simulink model "EDIF_start_up_v03"  (R2021b)
settings: Solver=FixedStepDiscrete  StartTime=0.0  StopTime=Inf  FixedStep=Ts  RelTol=1e-3  EnableMultiTasking=on
undefined symbols (not defined in the file or in its folder): Down, GPTRIP1SEL, Ts, TZ1, Up
libraries: c280xlib x6, svdutilitieslib x4, c2837xDlib x3, c2802xlib x2, simulink_extras x2, simulink x1, c2000sensorslib x1
settings Model: ExtModeTrigDuration=8  Creator=whendrix  LastModifiedBy=whendrix
settings SolverCC: AlgebraicLoopSolver=TrustRegion  AutoInsertRateTranBlk=on
settings DataIOCC: ReturnWorkspaceOutputs=off
settings OptimizationCC: DefaultUnderspecifiedDataType=single  EnhancedBackFolding=on  PassReuseOutputArgsAs=Individual arguments  MaxStackSize=1024  OptimizeBlockOrder=speed  DifferentSizesBufferReuse=on  OptimizationCustomize=off  DenormalBehavior=FlushToZero  EfficientTunableParamExpr=on
settings DebuggingCC: ParameterOverflowMsg=warning  ParameterPrecisionLossMsg=none  ParameterTunabilityLossMsg=error  SFMachineParentedDataDiag=warning  ArithmeticOperatorsInVariantConditions=warning
settings HardwareCC: ProdBitPerChar=16  ProdBitPerInt=16  ProdBitPerPointer=32  ProdBitPerSizeT=32  ProdBitPerPtrDiffT=32  ProdLargestAtomicInteger=Integer  ProdLargestAtomicFloat=None  ProdWordSize=16  ProdLongLongMode=on  ProdHWDeviceType=Texas Instruments->C2000
settings SFSimCC: MATLABDynamicMemAlloc=off  CustomCodeUndefinedFunction=UseInterfaceOnly
settings RTWCC: Description=Embedded Coder  SystemTargetFile=ert.tlc  HardwareBoard=TI Delfino F28379D LaunchPad  TemplateMakefile=ert_default_tmf  Toolchain=Texas Instruments Code Composer Studio (C2000)  IncludeHyperlinkInReport=on
settings CodeAppCC: ForceParamTrailComments=on  IgnoreCustomStorageClasses=off  OperatorAnnotations=on  SimulinkDataObjDesc=on  SFDataObjDesc=on  InsertBlockDesc=on
settings ERTTargetCC: CodeReplacementLibrary=TI C28x  ExtModeTransport=4  ExtModeStaticAlloc=on  ExtModeMexFile=ext_xcp  ExtModeIntrfLevel=Level2 - Open

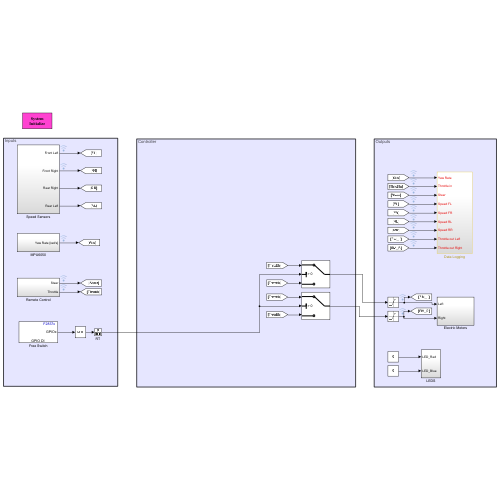
[thumbnail: Simulink's stored preview of the top-level diagram]
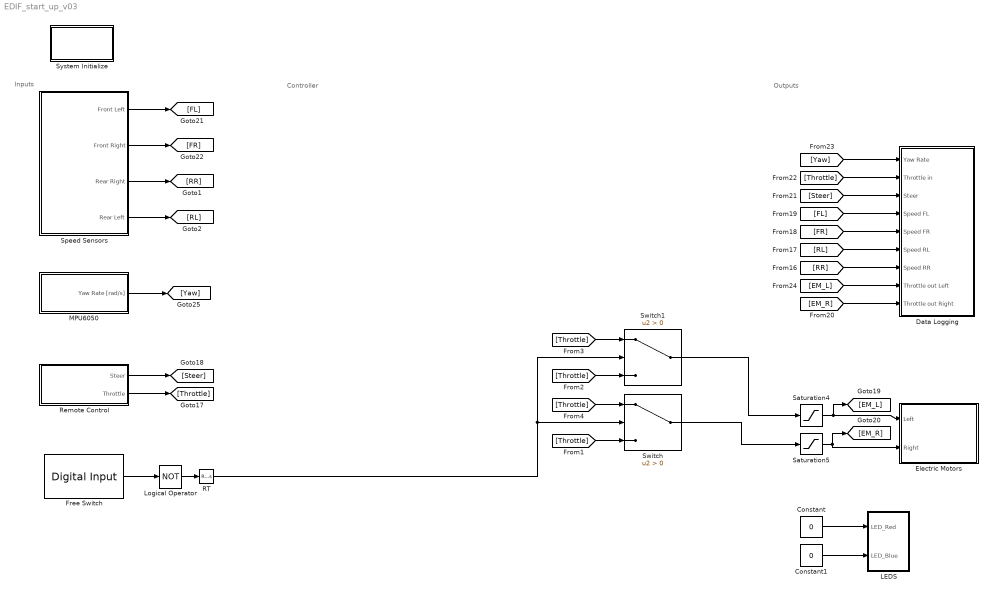
== system EDIF_start_up_v03 ==
  note: Controller
  note: Inputs
  note: Outputs
  Constant : Constant  Value=0
  Constant1 : Constant  Value=0
  Data Logging : Subsystem
  Electric Motors : Subsystem
  Free Switch : c2837xDlib/Digital Input  GPIO_Number=GPIO120~GPIO127  GPIO_Bit0=off  GPIO_Bit1=off  GPIO_Bit2=on  GPIO_Bit3=off  GPIO_Bit4=off  GPIO_Bit5=off  GPIO_Bit6=off  GPIO_Bit7=off  sampleTime=0.1  dataType=auto  GPIO_Bit0_Qualification=Sync to SYSCLKOUT  GPIO_Bit1_Qualification=Sync to SYSCLKOUT  GPIO_Bit2_Qualification=Sync to SYSCLKOUT  GPIO_Bit3_Qualification=Sync to SYSCLKOUT  GPIO_Bit4_Qualification=Sync to SYSCLKOUT  GPIO_Bit5_Qualification=Sync to SYSCLKOUT  GPIO_Bit6_Qualification=Sync to SYSCLKOUT  GPIO_Bit7_Qualification=Sync to SYSCLKOUT  Qualification_Period=-1
      settings: SourceProductBaseCode=TIC2000
  LEDS : Subsystem
  Logical Operator : Logic  Operator=NOT  AllPortsSameDT=off  OutDataTypeStr=boolean
  MPU6050 : Subsystem
  RT : RateTransition  OutPortSampleTime=0.005
  Remote Control : Subsystem
  Saturation4 : Saturate  UpperLimit=100  LowerLimit=20
  Saturation5 : Saturate  UpperLimit=100  LowerLimit=20
  Speed Sensors : Subsystem
  Switch : Switch  Criteria=u2 > Threshold  OutDataTypeStr=single
  Switch1 : Switch  Criteria=u2 > Threshold  OutDataTypeStr=single
  System Initialize : Subsystem  mask(System Initialize){ShowInLibBrowser=0}
      mask prompts: ShowInLibBrowser "Simulink:masks:CustCodeMaskParam1_MP"
      settings: CopyFcn=cccopyfcn(gcb)  OpenFcn=ccopenfcn('System Initialize Function')
      mask Help: eval('feval(''rtwprivate'',''rtwhelpview'',''rtw_sys_initialize_block'')');
      mask Display: disp('System\nInitialize');
  wires:
  MPU6050/1(Yaw Rate [rad/s]) -> [Yaw]
  Speed Sensors/1(Front Left) -> [FL]
  Saturation5/1 -> [EM_R], Electric Motors/2(Right)
  Saturation4/1 -> [EM_L], Electric Motors/1(Left)
  Speed Sensors/2(Front Right) -> [FR]
  Constant/1 -> LEDS/1(LED_Red)
  Remote Control/1(Steer) -> [Steer]
  [Yaw] -> Data Logging/1(Yaw Rate)
  [Throttle] -> Data Logging/2(Throttle in)
  [Steer] -> Data Logging/3(Steer)
  [FL] -> Data Logging/4(Speed FL)
  [FR] -> Data Logging/5(Speed FR)
  [RL] -> Data Logging/6(Speed RL)
  [RR] -> Data Logging/7(Speed RR)
  [EM_L] -> Data Logging/8(Throttle out Left)
  [EM_R] -> Data Logging/9(Throttle out Right)
  Speed Sensors/3(Rear Right) -> [RR]
  Speed Sensors/4(Rear Left) -> [RL]
  Remote Control/2(Throttle) -> [Throttle]
  Switch/1 -> Saturation5/1
  Switch1/1 -> Saturation4/1
  RT/1 -> Switch1/2, Switch/2
  [Throttle] -> Switch/3
  [Throttle] -> Switch1/3
  Logical Operator/1 -> RT/1
  Constant1/1 -> LEDS/2(LED_Blue)
  Free Switch/1 -> Logical Operator/1
  [Throttle] -> Switch1/1
  [Throttle] -> Switch/1

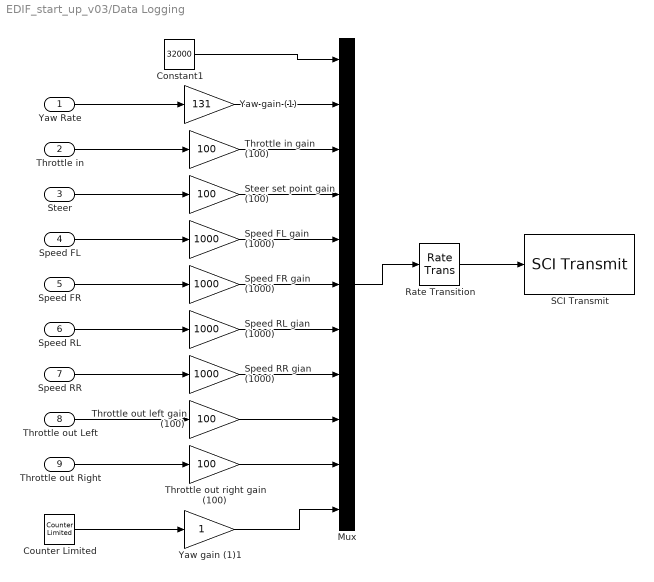
== system EDIF_start_up_v03/Data Logging ==
  Yaw Rate : Inport
  Throttle in : Inport  Port=2
  Steer : Inport  Port=3
  Speed FL : Inport  Port=4
  Speed FR : Inport  Port=5
  Speed RL : Inport  Port=6
  Speed RR : Inport  Port=7
  Throttle out Left : Inport  Port=8
  Throttle out Right : Inport  Port=9
  Constant1 : Constant  Value=32000  OutDataTypeStr=int16  SampleTime=0.005
  Counter Limited : simulink/Sources/Counter Limited  uplimit=30000  tsamp=Ts
  Mux : Mux  Inputs=11
  Rate Transition : RateTransition  OutPortSampleTime=0.01
  SCI Transmit : c280xlib/SCI Transmit  sciModule=B  dataHead=''  dataTail=''  postInterrupt=off  numFifo=1
  Speed FL gain (1000) : Gain  Gain=1000  OutDataTypeStr=int16
  Speed FR gain (1000) : Gain  Gain=1000  OutDataTypeStr=int16
  Speed RL gian (1000) : Gain  Gain=1000  OutDataTypeStr=int16
  Speed RR gian (1000) : Gain  Gain=1000  OutDataTypeStr=int16
  Steer set point gain (100) : Gain  Gain=100  OutDataTypeStr=int16
  Throttle in gain (100) : Gain  Gain=100  OutDataTypeStr=int16
  Throttle out left gain (100) : Gain  Gain=100  OutDataTypeStr=int16
  Throttle out right gain (100) : Gain  Gain=100  OutDataTypeStr=int16
  Yaw gain (1) : Gain  Gain=131  OutDataTypeStr=int16
  Yaw gain (1)1 : Gain  OutDataTypeStr=int16
  wires:
  Rate Transition/1 -> SCI Transmit/1
  Throttle out Left/1 -> Throttle out left gain (100)/1
  Speed RR/1 -> Speed RR gian (1000)/1
  Speed FR/1 -> Speed FR gain (1000)/1
  Speed RL/1 -> Speed RL gian (1000)/1
  Speed FL/1 -> Speed FL gain (1000)/1
  Throttle out Right/1 -> Throttle out right gain (100)/1
  Yaw Rate/1 -> Yaw gain (1)/1
  Throttle in/1 -> Throttle in gain (100)/1
  Steer/1 -> Steer set point gain (100)/1
  Throttle out right gain (100)/1 -> Mux/10
  Throttle out left gain (100)/1 -> Mux/9
  Speed RR gian (1000)/1 -> Mux/8
  Speed RL gian (1000)/1 -> Mux/7
  Speed FR gain (1000)/1 -> Mux/6
  Speed FL gain (1000)/1 -> Mux/5
  Steer set point gain (100)/1 -> Mux/4
  Throttle in gain (100)/1 -> Mux/3
  Yaw gain (1)/1 -> Mux/2
  Mux/1 -> Rate Transition/1
  Constant1/1 -> Mux/1
  Counter Limited/1 -> Yaw gain (1)1/1
  Yaw gain (1)1/1 -> Mux/11

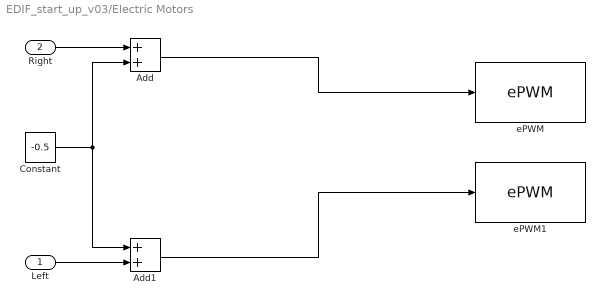
== system EDIF_start_up_v03/Electric Motors ==
  Left : Inport
  Right : Inport  Port=2
  Add : Sum
  Add1 : Sum
  Constant : Constant  Value=-0.5
  ePWM : c2802xlib/ePWM  PwmType=C2000_Type4  useModule=ePWM4  ePWMxLINKTBPRD=Not Linked  periodUnits=Clock cycles  timerSource=Specify via dialog  timerPeriod_clk=2000  timerPeriod_sec=0.0001  tbshadow=Counter equals to zero  countingMode=Up-Down  phaseActiveEnable=Disable  phaseDirection=Count down after sync  phaseActive=0  synchronizationEnable=off  dcaevt1Sync=off  dcbevt1Sync=off  synchronizationOption=Disable  perSynchronizationOption=Counter equals to period (CTR=PRD)  clockPrescale=1  HSclockPrescale=1  enswap=off  ePWMxAStatus=on  ePWMxAactionLogic1=Set  ePWMxAactionLogic2=Clear  ePWMxAactionLogic3=Clear  ePWMxAactionLogic4=Set  ePWMxAactionLogic5=Do nothing  ePWMxAactionLogic6=Do nothing  ePWMxACSFenable=off  ePWMxACSFvalue=Forcing disable  ePWMxASFreload=Zero  ePWMxBStatus=off  ePWMxBactionLogic1=Set  ePWMxBactionLogic2=Clear  ePWMxBactionLogic3=Do nothing  ePWMxBactionLogic4=Do nothing  ePWMxBactionLogic5=Clear  ePWMxBactionLogic6=Set  ePWMxBCSFenable=off  ePWMxBCSFvalue=Forcing disable  ePWMxBSFreload=Zero  ePWNxBOutWay=off  ePWMxLINKCMPA=Not Linked  CMPAUnits=Percentages  CMPASource=Input port  CMPAValue_per=50  CMPAValue_clk=32000  enCMPAshadow=Counter equals to zero (CTR=Zero)  ePWMxLINKCMPB=Not Linked  CMPBUnits=Clock cycles  CMPBSource=Specify via dialog  CMPBValue_per=50  CMPBValue_clk=32000  enCMPBshadow=Counter equals to zero (CTR=Zero)  ePWMxLINKCMPC=Not Linked  CMPCUnits=Clock cycles  CMPCSource=Specify via dialog  CMPCValue_per=50  CMPCValue_clk=32000  enCMPCshadow=Counter equals to zero (CTR=Zero)  ePWMxLINKCMPD=Not Linked  CMPDUnits=Clock cycles  CMPDSource=Specify via dialog  CMPDValue_per=50  CMPDValue_clk=32000  enCMPDshadow=Counter equals to zero (CTR=Zero)  enableDBePWMxA=off  enableDBePWMxB=off  enhalfcycle=off  DBpolarity=Active high (AH)  DBedgeDelay=Positive  DBSource_ePWMxA=ePWMxA  DBSource_ePWMxB=ePWMxA  DBPeriodUnits=Clock cycles  DBperiodSource=Specify via dialog  REDperiod=0  FEDperiod=0  REDperiod_sec=0  FEDperiod_sec=0  LoadModeDBRED=Immediate without using shadow  LoadModeDBFED=Immediate without using shadow  adcstartModuleA=off  adcrequestEventA=First event  adcstartEventA=Digital Compare Module A Event 1 start of conversion (DCAEVT1.soc)  adcstartEventA_type2=Counter equals to zero (CTR=Zero)  adcstartModuleB=off  adcrequestEventB=First event  adcstartEventB=Counter equals to zero (CTR=Zero)  adcstartEventB_type2=Counter equals to zero (CTR=Zero)  intEn=off  intPrd=First event  intSel=Counter equals to zero (CTR=Zero)  intSel_type2=Counter equals to zero (CTR=Zero)  hrpe=off  enHRPWM=off  HRPWM_LoadMode=Counter equals to period (CTR=PRD)  HRPWM_CTLMode=Duty or Period control mode  HRPWM_EDGMode=Both edge  hrpeb=off  enHRPWMB=off  HRPWM_LoadModeB=Counter equals to zero (CTR=ZERO)  HRPWM_CTLModeB=Duty or Period control mode  HRPWM_EDGModeB=Both edge  enHRDBRED=off  enHRDBFED=off  enSFO=on  enautoconv=on  chopperEnable=off  chopperFrequency=1  chopperFirstwidth=1  chopperDuty=12.5%  tripZonesource=Specify via dialog  tzselOSHT1=off  tzselOSHT2=off  tzselOSHT3=off  tzselOSHDCAEV1=off  tzselOSHDCBEV1=off  tzselCBC1=off  tzselCBC2=off  tzselCBC3=off  tzselCBCDCAEV2=off  tzselCBCDCBEV2=off  tzselOSHT4=off  tzselOSHT5=off  tzselOSHT6=off  tzselCBC4=off  tzselCBC5=off  tzselCBC6=off  enTzOstIntr=off  enTzCbcIntr=off  enTzDCAEVT1Intr=off  enTzDCAEVT2Intr=off  enTzDCBEVT1Intr=off  enTzDCBEVT2Intr=off  ePWMxAforced=No action  ePWMxBforced=No action  DCAEVT1forced=No action  DCBEVT1forced=No action  DCAEVT2forced=No action  DCBEVT2forced=No action  dcah=Trip Zone 1 input (TZ1)  dcal=Trip Zone 2 input (TZ2)  dcbh=Trip Zone 1 input (TZ1)  dcbl=Trip Zone 2 input (TZ2)  dcah_type2=GPTRIP1SEL/(TZ1)  dcal_type2=GPTRIP1SEL/(TZ1)  dcbh_type2=GPTRIP1SEL/(TZ1)  dcbl_type2=GPTRIP1SEL/(TZ1)  gendcaevt1=Event disabled  gendcaevt2=Event disabled  gendcbevt1=Event disabled  gendcbevt2=Event disabled  dcaevt1src=DCAEVT1 with sync  dcaevt2src=DCAEVT2 with sync  dcbevt1src=DCBEVT1 with sync  dcbevt2src=DCBEVT2 with sync  pulsesel=Counter equals to zero (CTR=Zero)  blankinv=off  blankoffset=0  blankwidth=0  evsrcsel=Filtered version of DCAEVT1 (DCAEVT1FILT)  encape=off
  ePWM1 : c2802xlib/ePWM  PwmType=C2000_Type4  useModule=ePWM5  ePWMxLINKTBPRD=Not Linked  periodUnits=Clock cycles  timerSource=Specify via dialog  timerPeriod_clk=2000  timerPeriod_sec=0.0001  tbshadow=Counter equals to zero  countingMode=Up-Down  phaseActiveEnable=Disable  phaseDirection=Count down after sync  phaseActive=0  synchronizationEnable=off  dcaevt1Sync=off  dcbevt1Sync=off  synchronizationOption=Disable  perSynchronizationOption=Counter equals to period (CTR=PRD)  clockPrescale=1  HSclockPrescale=1  enswap=off  ePWMxAStatus=on  ePWMxAactionLogic1=Set  ePWMxAactionLogic2=Clear  ePWMxAactionLogic3=Clear  ePWMxAactionLogic4=Set  ePWMxAactionLogic5=Do nothing  ePWMxAactionLogic6=Do nothing  ePWMxACSFenable=off  ePWMxACSFvalue=Forcing disable  ePWMxASFreload=Zero  ePWMxBStatus=off  ePWMxBactionLogic1=Set  ePWMxBactionLogic2=Clear  ePWMxBactionLogic3=Do nothing  ePWMxBactionLogic4=Do nothing  ePWMxBactionLogic5=Clear  ePWMxBactionLogic6=Set  ePWMxBCSFenable=off  ePWMxBCSFvalue=Forcing disable  ePWMxBSFreload=Zero  ePWNxBOutWay=off  ePWMxLINKCMPA=Not Linked  CMPAUnits=Percentages  CMPASource=Input port  CMPAValue_per=50  CMPAValue_clk=32000  enCMPAshadow=Counter equals to zero (CTR=Zero)  ePWMxLINKCMPB=Not Linked  CMPBUnits=Clock cycles  CMPBSource=Specify via dialog  CMPBValue_per=50  CMPBValue_clk=32000  enCMPBshadow=Counter equals to zero (CTR=Zero)  ePWMxLINKCMPC=Not Linked  CMPCUnits=Clock cycles  CMPCSource=Specify via dialog  CMPCValue_per=50  CMPCValue_clk=32000  enCMPCshadow=Counter equals to zero (CTR=Zero)  ePWMxLINKCMPD=Not Linked  CMPDUnits=Clock cycles  CMPDSource=Specify via dialog  CMPDValue_per=50  CMPDValue_clk=32000  enCMPDshadow=Counter equals to zero (CTR=Zero)  enableDBePWMxA=off  enableDBePWMxB=off  enhalfcycle=off  DBpolarity=Active high (AH)  DBedgeDelay=Positive  DBSource_ePWMxA=ePWMxA  DBSource_ePWMxB=ePWMxA  DBPeriodUnits=Clock cycles  DBperiodSource=Specify via dialog  REDperiod=0  FEDperiod=0  REDperiod_sec=0  FEDperiod_sec=0  LoadModeDBRED=Immediate without using shadow  LoadModeDBFED=Immediate without using shadow  adcstartModuleA=off  adcrequestEventA=First event  adcstartEventA=Digital Compare Module A Event 1 start of conversion (DCAEVT1.soc)  adcstartEventA_type2=Counter equals to zero (CTR=Zero)  adcstartModuleB=off  adcrequestEventB=First event  adcstartEventB=Counter equals to zero (CTR=Zero)  adcstartEventB_type2=Counter equals to zero (CTR=Zero)  intEn=off  intPrd=First event  intSel=Counter equals to zero (CTR=Zero)  intSel_type2=Counter equals to zero (CTR=Zero)  hrpe=off  enHRPWM=off  HRPWM_LoadMode=Counter equals to period (CTR=PRD)  HRPWM_CTLMode=Duty or Period control mode  HRPWM_EDGMode=Both edge  hrpeb=off  enHRPWMB=off  HRPWM_LoadModeB=Counter equals to zero (CTR=ZERO)  HRPWM_CTLModeB=Duty or Period control mode  HRPWM_EDGModeB=Both edge  enHRDBRED=off  enHRDBFED=off  enSFO=on  enautoconv=on  chopperEnable=off  chopperFrequency=1  chopperFirstwidth=1  chopperDuty=12.5%  tripZonesource=Specify via dialog  tzselOSHT1=off  tzselOSHT2=off  tzselOSHT3=off  tzselOSHDCAEV1=off  tzselOSHDCBEV1=off  tzselCBC1=off  tzselCBC2=off  tzselCBC3=off  tzselCBCDCAEV2=off  tzselCBCDCBEV2=off  tzselOSHT4=off  tzselOSHT5=off  tzselOSHT6=off  tzselCBC4=off  tzselCBC5=off  tzselCBC6=off  enTzOstIntr=off  enTzCbcIntr=off  enTzDCAEVT1Intr=off  enTzDCAEVT2Intr=off  enTzDCBEVT1Intr=off  enTzDCBEVT2Intr=off  ePWMxAforced=No action  ePWMxBforced=No action  DCAEVT1forced=No action  DCBEVT1forced=No action  DCAEVT2forced=No action  DCBEVT2forced=No action  dcah=Trip Zone 1 input (TZ1)  dcal=Trip Zone 2 input (TZ2)  dcbh=Trip Zone 1 input (TZ1)  dcbl=Trip Zone 2 input (TZ2)  dcah_type2=GPTRIP1SEL/(TZ1)  dcal_type2=GPTRIP1SEL/(TZ1)  dcbh_type2=GPTRIP1SEL/(TZ1)  dcbl_type2=GPTRIP1SEL/(TZ1)  gendcaevt1=Event disabled  gendcaevt2=Event disabled  gendcbevt1=Event disabled  gendcbevt2=Event disabled  dcaevt1src=DCAEVT1 with sync  dcaevt2src=DCAEVT2 with sync  dcbevt1src=DCBEVT1 with sync  dcbevt2src=DCBEVT2 with sync  pulsesel=Counter equals to zero (CTR=Zero)  blankinv=off  blankoffset=0  blankwidth=0  evsrcsel=Filtered version of DCAEVT1 (DCAEVT1FILT)  encape=off
  wires:
  Right/1 -> Add/1
  Constant/1 -> Add/2, Add1/1
  Left/1 -> Add1/2
  Add/1 -> ePWM/1
  Add1/1 -> ePWM1/1

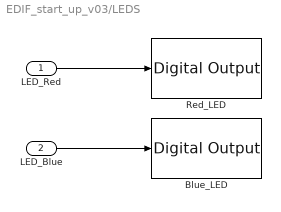
== system EDIF_start_up_v03/LEDS ==
  LED_Red : Inport
  LED_Blue : Inport  Port=2
  Blue_LED : c2837xDlib/Digital Output  GPIO_Number=GPIO24~GPIO31  GPIO_Bit0=off  GPIO_BIT0_Toggle=off  GPIO_Bit1=off  GPIO_BIT1_Toggle=off  GPIO_Bit2=off  GPIO_BIT2_Toggle=off  GPIO_Bit3=off  GPIO_BIT3_Toggle=off  GPIO_Bit4=off  GPIO_BIT4_Toggle=off  GPIO_Bit5=off  GPIO_BIT5_Toggle=off  GPIO_Bit6=off  GPIO_BIT6_Toggle=off  GPIO_Bit7=on  GPIO_BIT7_Toggle=off
      settings: SourceProductBaseCode=TIC2000
  Red_LED : c2837xDlib/Digital Output  GPIO_Number=GPIO32~GPIO39  GPIO_Bit0=off  GPIO_BIT0_Toggle=off  GPIO_Bit1=off  GPIO_BIT1_Toggle=off  GPIO_Bit2=on  GPIO_BIT2_Toggle=off  GPIO_Bit3=off  GPIO_BIT3_Toggle=off  GPIO_Bit4=off  GPIO_BIT4_Toggle=off  GPIO_Bit5=off  GPIO_BIT5_Toggle=off  GPIO_Bit6=off  GPIO_BIT6_Toggle=off  GPIO_Bit7=off  GPIO_BIT7_Toggle=off
      settings: SourceProductBaseCode=TIC2000
  wires:
  LED_Red/1 -> Red_LED/1
  LED_Blue/1 -> Blue_LED/1

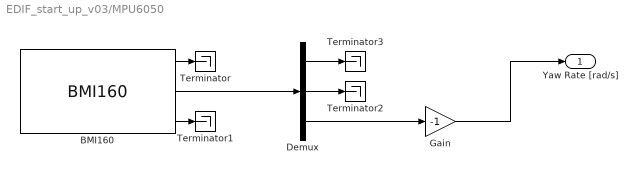
== system EDIF_start_up_v03/MPU6050 ==
  BMI160 : c2000sensorslib/BMI160  I2CModule=I2C_A  I2CAddress=0x69  IsActiveInterrupt=off  InterruptPin=INT1  EnableSecondaryMag=on  MagnetometerI2CAddress=0x13  BitRate=1000000  IsActiveAccel=on  IsActiveGyro=on  IsActiveMag=on  IsActiveTemperature=off  IsAccelStatus=off  IsGyroStatus=off  IsMagStatus=off  DataType=single  SampleTime=-1  AccelerationRange=+/- 2g  AccelerometerODR=200 Hz  IsEnableAccelLowPassFilter=off  AccelerometerFilterMode=Normal  GyroscopeRange=125 dps  GyroscopeODR=200 Hz  IsEnableGyroLowPassFilter=off  GyroscopeFilterMode=Normal  MagnetometerODR=25 Hz
      settings: SourceProductBaseCode=TIC2000
  Demux : Demux  Outputs=3
  Gain : Gain  Gain=-1
  Terminator{,1..3} (4 alike) : Terminator
  Yaw Rate [rad/s] : Outport  VectorParamsAs1DForOutWhenUnconnected=off
  wires:
  BMI160/1 -> Terminator/1
  BMI160/3 -> Terminator1/1
  BMI160/2 -> Demux/1
  Demux/2 -> Terminator2/1
  Demux/3 -> Gain/1
  Demux/1 -> Terminator3/1
  Gain/1 -> Yaw Rate [rad/s]/1

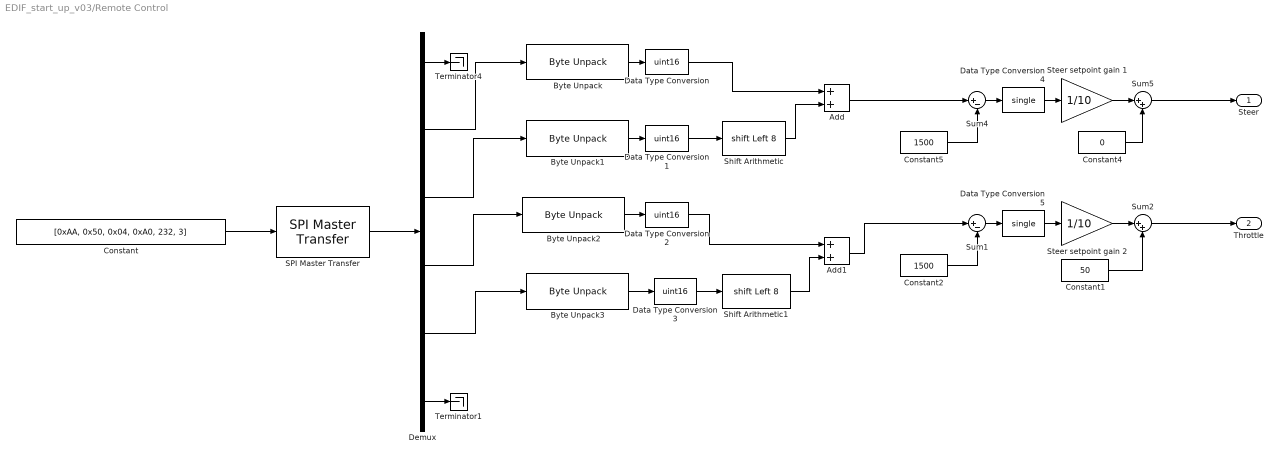
== system EDIF_start_up_v03/Remote Control ==
  Add : Sum
  Add1 : Sum
  Byte Unpack{,1..3} (4 alike) : svdutilitieslib/Byte Unpack  dimensions={[1]}  datatypes={'uint16'}  byteAlign=2  blockPlatform=tic2000
      settings: SourceProductBaseCode=ANDROID,ARDUINO,ML_ARDUINO,ECCORTEXA,ECCORTEXR,SC_BEAGLEBONE_BLUE,EC_FREEDOM_BOARD,EC_FRDM_K64F,INTEL_BLOCKSET,MICROBIT,NUCLEO,NVIDIA,PX4AUTOPILOTS,RASPPIIO,STMICRODIS,TIC2000,XILINX_BLOCKSET
  Constant : Constant  Value=[0xAA, 0x50, 0x04, 0xA0, 232, 3]  OutDataTypeStr=uint16
  Constant1 : Constant  Value=50  OutDataTypeStr=single  SampleTime=0.005
  Constant2 : Constant  Value=1500  OutDataTypeStr=single  SampleTime=Ts
  Constant4 : Constant  Value=0  OutDataTypeStr=single  SampleTime=0.005
  Constant5 : Constant  Value=1500  OutDataTypeStr=single  SampleTime=Ts
  Data Type Conversion{,1..3} (4 alike) : DataTypeConversion  OutDataTypeStr=uint16
  Data Type Conversion4 : DataTypeConversion  OutDataTypeStr=single
  Data Type Conversion5 : DataTypeConversion  OutDataTypeStr=single
  Demux : Demux  Outputs=6
  SPI Master Transfer : c280xlib/SPI Master Transfer  SPISelect=SPI_A  ClockPolarity=Rising_edge  ClockPhase=No_delay  SPIModule=uint32(0)  Mode=Master  BusSpeed=uint32(1000000)  FirstBitToTransfer=Most significant bit (MSB)  ClockMode=0  BlockFunction=Transfer  EnableRegisterAddress=off  RegisterAddress=0  OutputDataType=int8  OutputDataLength=1  DataBits=8  UseCustomSSPin=Explicit GPIO calls  ActiveLowSSPin=Active low  Pin=61
      settings: SourceProductBaseCode=TIC2000
  Shift Arithmetic : ArithShift  BitShiftNumber=8  BitShiftDirection=Left
  Shift Arithmetic1 : ArithShift  BitShiftNumber=8  BitShiftDirection=Left
  Steer setpoint gain 1 : Gain  Gain=1/10  OutDataTypeStr=single
  Steer setpoint gain 2 : Gain  Gain=1/10  OutDataTypeStr=single
  Sum1 : Sum  Inputs=|+-
  Sum2 : Sum  Inputs=|++
  Sum4 : Sum  Inputs=|+-
  Sum5 : Sum  Inputs=|++
  Terminator1 : Terminator
  Terminator4 : Terminator
  Steer : Outport  VectorParamsAs1DForOutWhenUnconnected=off
  Throttle : Outport  Port=2  VectorParamsAs1DForOutWhenUnconnected=off
  wires:
  Constant/1 -> SPI Master Transfer/1
  SPI Master Transfer/1 -> Demux/1
  Byte Unpack/1 -> Data Type Conversion/1
  Byte Unpack3/1 -> Data Type Conversion3/1
  Add/1 -> Sum4/1
  Byte Unpack1/1 -> Data Type Conversion1/1
  Byte Unpack2/1 -> Data Type Conversion2/1
  Shift Arithmetic/1 -> Add/2
  Shift Arithmetic1/1 -> Add1/2
  Data Type Conversion/1 -> Add/1
  Data Type Conversion1/1 -> Shift Arithmetic/1
  Data Type Conversion2/1 -> Add1/1
  Data Type Conversion3/1 -> Shift Arithmetic1/1
  Constant5/1 -> Sum4/2
  Constant4/1 -> Sum5/2
  Steer setpoint gain 1/1 -> Sum5/1
  Sum4/1 -> Data Type Conversion4/1
  Sum1/1 -> Data Type Conversion5/1
  Steer setpoint gain 2/1 -> Sum2/1
  Constant1/1 -> Sum2/2
  Constant2/1 -> Sum1/2
  Sum2/1 -> Throttle/1
  Data Type Conversion4/1 -> Steer setpoint gain 1/1
  Data Type Conversion5/1 -> Steer setpoint gain 2/1
  Add1/1 -> Sum1/1
  Demux/6 -> Terminator1/1
  Sum5/1 -> Steer/1
  Demux/2 -> Byte Unpack/1
  Demux/1 -> Terminator4/1
  Demux/3 -> Byte Unpack1/1
  Demux/4 -> Byte Unpack2/1
  Demux/5 -> Byte Unpack3/1

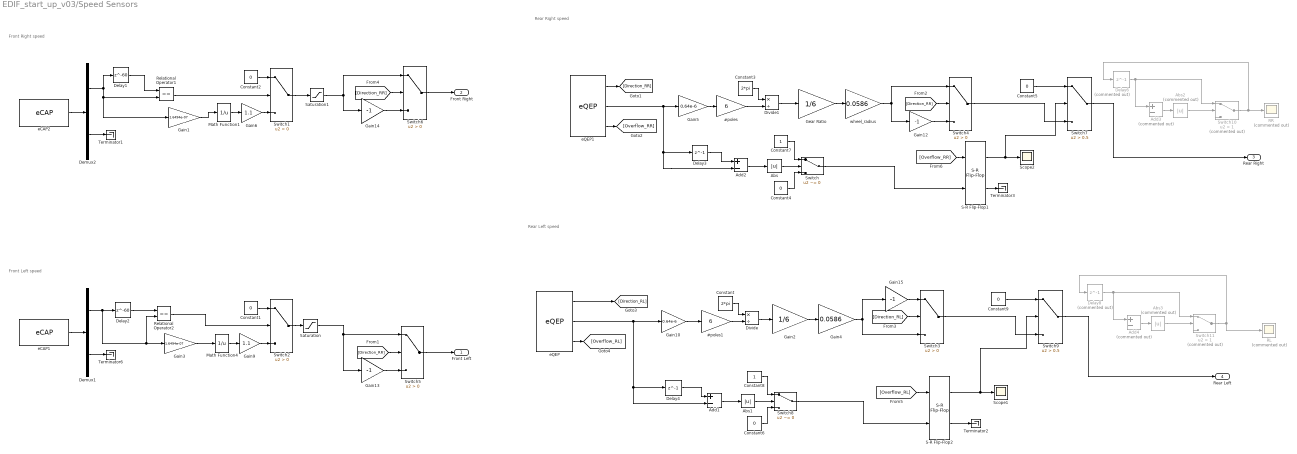
== system EDIF_start_up_v03/Speed Sensors ==
  note: Front Right speed
  note: Front Left speed
  note: Rear Right speed
  note: Rear Left speed
  #poles : Gain  Gain=6
  #poles1 : Gain  Gain=6
  Abs : Abs
  Abs1 : Abs
  Abs2 : Abs  Commented=on
  Abs3 : Abs  Commented=on
  Add1 : Sum  Inputs=+-  OutDataTypeStr=single
  Add2 : Sum  Inputs=+-  OutDataTypeStr=single
  Add3 : Sum  Commented=on  Inputs=+-
  Add4 : Sum  Commented=on  Inputs=+-
  Constant : Constant  Value=2*pi
  Constant1 : Constant  Value=0  OutDataTypeStr=int8  SampleTime=0.005
  Constant2 : Constant  Value=0  OutDataTypeStr=int8  SampleTime=0.005
  Constant3 : Constant  Value=2*pi
  Constant4 : Constant  Value=0  OutDataTypeStr=boolean
  Constant5 : Constant  Value=0
  Constant6 : Constant  Value=0  OutDataTypeStr=boolean
  Constant7 : Constant  OutDataTypeStr=boolean
  Constant8 : Constant  OutDataTypeStr=boolean
  Constant9 : Constant  Value=0
  Delay1 : Delay  DelayLength=60
  Delay2 : Delay  DelayLength=60
  Delay3 : Delay  DelayLength=1
  Delay4 : Delay  DelayLength=1
  Delay6 : Delay  Commented=on  DelayLength=1
  Delay8 : Delay  Commented=on  DelayLength=1
  Demux1 : Demux  Outputs=2
  Demux2 : Demux  Outputs=2
  Divide : Product  Inputs=*/
  Divide1 : Product  Inputs=*/
  Gain1 : Gain  Gain=1.6494e-07
  Gain10 : Gain  Gain=0.64e-6
  Gain{12..15} (4 alike) : Gain  Gain=-1
  Gain2 : Gain  Gain=1/6
  Gain3 : Gain  Gain=1.6494e-07
  Gain4 : Gain  Gain=0.0586
  Gain5 : Gain  Gain=0.64e-6
  Gain6 : Gain  Gain=1.1
  Gain9 : Gain  Gain=1.1
  Gear Ratio : Gain  Gain=1/6
  Math Function1 : Math  Operator=reciprocal  SignedPower=on  SaturateOnIntegerOverflow=on
  Math Function4 : Math  Operator=reciprocal  SignedPower=on  SaturateOnIntegerOverflow=on
  RL : Scope  Commented=on
  RR : Scope  Commented=on
  Relational Operator1 : RelationalOperator  Operator===  OutDataTypeStr=boolean  RndMeth=Nearest
  Relational Operator2 : RelationalOperator  Operator===  OutDataTypeStr=boolean  RndMeth=Nearest
  S-R Flip-Flop1 : simulink_extras/Flip Flops/S-R Flip-Flop  initial_condition=1
  S-R Flip-Flop2 : simulink_extras/Flip Flops/S-R Flip-Flop  initial_condition=1
  Saturation : Saturate  UpperLimit=40/3.6  LowerLimit=0
  Saturation1 : Saturate  UpperLimit=40/3.6  LowerLimit=0
  Scope1 : Scope
  Scope2 : Scope
  Switch : Switch  Criteria=u2 ~= 0  Threshold=10
  Switch{1..6} (6 alike) : Switch  Criteria=u2 > Threshold  OutDataTypeStr=single
  Switch10 : Switch  Commented=on  Criteria=u2 > Threshold  Threshold=1
  Switch11 : Switch  Commented=on  Criteria=u2 > Threshold  Threshold=1
  Switch7 : Switch  Criteria=u2 > Threshold  Threshold=0.5  OutDataTypeStr=single
  Switch8 : Switch  Criteria=u2 ~= 0  Threshold=10
  Switch9 : Switch  Criteria=u2 > Threshold  Threshold=0.5  OutDataTypeStr=single
  Terminator{1..3,6} (4 alike) : Terminator
  eCAP1 : c280xlib/eCAP  operatingMode=eCAP  selectCAPx=eCAP1  offsetValue=0  counterSynIn=off  enableCounter=off  syncOutput=CTR=PRD  sampleTime=Ts  eventPrescaler=0  selectMode=Continuous  enableOneShot=off  stopValue=Capture Event 2  resetEv1Ts=on  ev1Polarity=Rising Edge  resetEv2Ts=on  ev2Polarity=Falling Edge  resetEv3Ts=off  ev3Polarity=Rising Edge  resetEv4Ts=off  ev4Polarity=Rising Edge  tSCntrDataType=uint32  capEvFlag=off  capFlagDataType=uint16  overFlowFlag=off  overFlowFlagDataType=uint16  periodUnit=Seconds  periodSource=Specify via dialog  waveformPeriod=0.001  dutyUnit=Percentages  dutySource=Specify via dialog  dutyCycle=50  outputPolarity=Active High  enableCEVT1Int=off  enableCEVT2Int=on  enableCEVT3Int=off  enableCEVT4Int=off  enableCTROVFInt=off  enablePRDInt=off  enableCMPInt=off
      settings: SourceProductBaseCode=TIC2000
  eCAP2 : c280xlib/eCAP  operatingMode=eCAP  selectCAPx=eCAP2  offsetValue=0  counterSynIn=off  enableCounter=off  syncOutput=CTR=PRD  sampleTime=Ts  eventPrescaler=0  selectMode=Continuous  enableOneShot=off  stopValue=Capture Event 2  resetEv1Ts=on  ev1Polarity=Rising Edge  resetEv2Ts=on  ev2Polarity=Falling Edge  resetEv3Ts=off  ev3Polarity=Rising Edge  resetEv4Ts=off  ev4Polarity=Rising Edge  tSCntrDataType=uint32  capEvFlag=off  capFlagDataType=uint16  overFlowFlag=off  overFlowFlagDataType=uint16  periodUnit=Seconds  periodSource=Specify via dialog  waveformPeriod=0.001  dutyUnit=Percentages  dutySource=Specify via dialog  dutyCycle=50  outputPolarity=Active High  enableCEVT1Int=off  enableCEVT2Int=on  enableCEVT3Int=off  enableCEVT4Int=off  enableCTROVFInt=off  enablePRDInt=off  enableCMPInt=off
      settings: SourceProductBaseCode=TIC2000
  eQEP : c280xlib/eQEP  useModule=eQEP1  pcInputmode=Quadrature-count  externalClockrate=2x resolution: Count the rising/falling edge  swapPolarityselection=Clockwise  qdfOutputport=on  qapPolarityselection=off  qbpPolarityselection=off  qipPolarityselection=off  qspPolarityselection=off  igatePolarityselection=off  sampleTime=Ts  pcOutputport=off  pcMaximumvalue=1  indexInitializationcheck=off  indexInitializationevent=Rising edge  strobeInitializationcheck=off  strobeInitializationevent=Rising edge  softwareInitializationcheck=off  softwareInitializationsource=Set to init value at start up  softwareInitializationmode=on  pcInitialvalue=2147483648  pcResetmode=Reset on an index event  ieloutputport=off  indexEventlatch=Rising edge  seloutputport=off  strobeEventlatch=Rising edge  pcefOutputport=off  enableEqepcapture=on  qctmrOutputport=off  qcprdOutputport=on  captureTimerprescaler=128  upEventprescaler=2  overflowErrorflag=on  directionErrorflag=off  captureTimerposition=On position counter read  unitTimerperiod=100000000  captureTimerlatch=off  capturePeriodlatch=off  positionCounterlatch=off  soenPolarityselection=off  spselPolarityselection=Index pin is used for sync output  compareValuesource=Specify via dialog  shadowMode=Load on QPOSCNT=0  compareValue=4294967295  syncOutputwidth=1  polaritySyncoutput=Active high  watchdogEnable=off  watchdogTimer=65535  outport1Datatype=auto  outport2Datatype=auto  outport3Datatype=auto  outport4Datatype=auto  outport5Datatype=auto  outport6Datatype=auto  outport7Datatype=auto  outport8Datatype=auto  outport9Datatype=auto  outport10Datatype=auto  outport11Datatype=auto  outport12Datatype=auto  eqepinterrupt_pce=off  eqepinterrupt_qpe=off  eqepinterrupt_qdc=off  eqepinterrupt_wto=off  eqepinterrupt_pcu=on  eqepinterrupt_pco=on  eqepinterrupt_pcr=off  eqepinterrupt_pcm=off  eqepinterrupt_sel=off  eqepinterrupt_iel=off  eqepinterrupt_uto=off  pheOutputport=off  watchdogOutputport=off  outport13Datatype=auto  outport14Datatype=auto
      settings: SourceProductBaseCode=TIC2000
  eQEP1 : c280xlib/eQEP  useModule=eQEP2  pcInputmode=Quadrature-count  externalClockrate=2x resolution: Count the rising/falling edge  swapPolarityselection=Clockwise  qdfOutputport=on  qapPolarityselection=off  qbpPolarityselection=off  qipPolarityselection=off  qspPolarityselection=off  igatePolarityselection=off  sampleTime=Ts  pcOutputport=off  pcMaximumvalue=1  indexInitializationcheck=off  indexInitializationevent=Rising edge  strobeInitializationcheck=off  strobeInitializationevent=Rising edge  softwareInitializationcheck=off  softwareInitializationsource=Set to init value at start up  softwareInitializationmode=on  pcInitialvalue=2147483648  pcResetmode=Reset on an index event  ieloutputport=off  indexEventlatch=Rising edge  seloutputport=off  strobeEventlatch=Rising edge  pcefOutputport=off  enableEqepcapture=on  qctmrOutputport=off  qcprdOutputport=on  captureTimerprescaler=128  upEventprescaler=2  overflowErrorflag=on  directionErrorflag=off  captureTimerposition=On position counter read  unitTimerperiod=100000000  captureTimerlatch=off  capturePeriodlatch=off  positionCounterlatch=off  soenPolarityselection=off  spselPolarityselection=Index pin is used for sync output  compareValuesource=Specify via dialog  shadowMode=Load on QPOSCNT=0  compareValue=4294967295  syncOutputwidth=1  polaritySyncoutput=Active high  watchdogEnable=off  watchdogTimer=65535  outport1Datatype=auto  outport2Datatype=auto  outport3Datatype=auto  outport4Datatype=auto  outport5Datatype=auto  outport6Datatype=auto  outport7Datatype=auto  outport8Datatype=auto  outport9Datatype=auto  outport10Datatype=auto  outport11Datatype=auto  outport12Datatype=auto  eqepinterrupt_pce=off  eqepinterrupt_qpe=off  eqepinterrupt_qdc=off  eqepinterrupt_wto=off  eqepinterrupt_pcu=on  eqepinterrupt_pco=on  eqepinterrupt_pcr=off  eqepinterrupt_pcm=off  eqepinterrupt_sel=off  eqepinterrupt_iel=off  eqepinterrupt_uto=off  pheOutputport=off  watchdogOutputport=off  outport13Datatype=auto  outport14Datatype=auto
      settings: SourceProductBaseCode=TIC2000
  wheel_radius : Gain  Gain=0.0586
  Front Left : Outport  VectorParamsAs1DForOutWhenUnconnected=off
  Front Right : Outport  Port=2  VectorParamsAs1DForOutWhenUnconnected=off
  Rear Right : Outport  Port=3  VectorParamsAs1DForOutWhenUnconnected=off
  Rear Left : Outport  Port=4  VectorParamsAs1DForOutWhenUnconnected=off
  wires:
  Demux1/2 -> Terminator6/1
  Demux1/1 -> Gain3/1, Relational Operator2/2, Delay2/1
  Delay2/1 -> Relational Operator2/1
  Relational Operator2/1 -> Switch2/2
  Constant1/1 -> Switch2/1
  Math Function4/1 -> Gain9/1
  eCAP1/1 -> Demux1/1
  Delay1/1 -> Relational Operator1/1
  Relational Operator1/1 -> Switch1/2
  Constant2/1 -> Switch1/1
  Math Function1/1 -> Gain6/1
  eCAP2/1 -> Demux2/1
  Switch2/1 -> Saturation/1
  Switch1/1 -> Saturation1/1
  eQEP/1 -> [Direction_RL]
  [Direction_RL] -> Switch3/2
  eQEP1/1 -> [Direction_RR]
  Divide/1 -> Gain2/1
  Gain2/1 -> Gain4/1
  Gear Ratio/1 -> wheel_radius/1
  Divide1/1 -> Gear Ratio/1
  eQEP1/2 -> Gain5/1, Add2/2, Delay3/1
  eQEP/2 -> Add1/2, Delay4/1, Gain10/1
  Constant/1 -> Divide/1
  Constant3/1 -> Divide1/1
  wheel_radius/1 -> Switch4/1, Gain12/1
  [Direction_RR] -> Switch4/2
  eQEP1/3 -> [Overflow_RR]
  Gain10/1 -> #poles1/1
  Gain5/1 -> #poles/1
  Switch5/1 -> Front Left/1
  Saturation/1 -> Switch5/1, Gain13/1
  [Direction_RR] -> Switch5/2
  [Direction_RR] -> Switch6/2
  Saturation1/1 -> Switch6/1, Gain14/1
  Switch6/1 -> Front Right/1
  Gain4/1 -> Switch3/3, Gain15/1
  Abs/1 -> Switch/2
  Add2/1 -> Abs/1
  Delay3/1 -> Add2/1
  [Overflow_RR] -> S-R Flip-Flop1/1
  Switch/1 -> S-R Flip-Flop1/2
  S-R Flip-Flop1/1 -> Switch7/2, Scope2/1
  S-R Flip-Flop1/2 -> Terminator3/1
  Constant4/1 -> Switch/3
  Constant7/1 -> Switch/1
  Switch4/1 -> Switch7/3
  Constant5/1 -> Switch7/1
  S-R Flip-Flop2/1 -> Switch9/2, Scope1/1
  Constant8/1 -> Switch8/1
  Add1/1 -> Abs1/1
  Delay4/1 -> Add1/1
  Abs1/1 -> Switch8/2
  [Overflow_RL] -> S-R Flip-Flop2/1
  Switch8/1 -> S-R Flip-Flop2/2
  S-R Flip-Flop2/2 -> Terminator2/1
  Constant6/1 -> Switch8/3
  Constant9/1 -> Switch9/1
  Switch3/1 -> Switch9/3
  eQEP/3 -> [Overflow_RL]
  Delay6/1 -> Add3/1, Switch10/1
  Switch10/1 -> RR/1, Delay6/1
  Abs2/1 -> Switch10/2
  Add3/1 -> Abs2/1
  Add4/1 -> Abs3/1
  Abs3/1 -> Switch11/2
  Delay8/1 -> Add4/1, Switch11/1
  Switch11/1 -> RL/1, Delay8/1
  #poles/1 -> Divide1/2
  #poles1/1 -> Divide/2
  Gain1/1 -> Math Function1/1
  Gain6/1 -> Switch1/3
  Gain3/1 -> Math Function4/1
  Gain9/1 -> Switch2/3
  Switch7/1 -> Rear Right/1
  Switch9/1 -> Rear Left/1
  Demux2/1 -> Delay1/1, Gain1/1, Relational Operator1/2
  Demux2/2 -> Terminator1/1
  Gain12/1 -> Switch4/3
  Gain14/1 -> Switch6/3
  Gain13/1 -> Switch5/3
  Gain15/1 -> Switch3/1

== system EDIF_start_up_v03/System Initialize ==
